simulink model "TEMA"  (R2017a)
settings: Solver=FixedStepAuto  StartTime=0.0  StopTime=10.0  FixedStep=0.01  RelTol=1e-3
libraries: MyEma x1
settings Model: Creator=alexandr.lanin  LastModifiedBy=alexandr.lanin

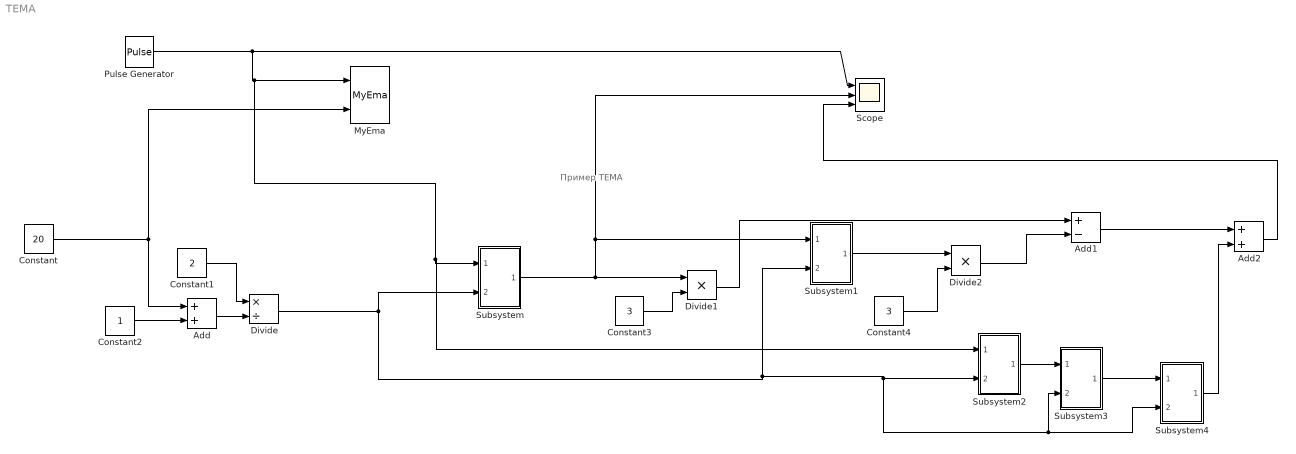
== system TEMA ==
  note: Пример TEMA
  Add : Sum
  Add1 : Sum  Inputs=+-
  Add2 : Sum
  Constant : Constant  Value=20
  Constant1 : Constant  Value=2
  Constant2 : Constant
  Constant3 : Constant  Value=3
  Constant4 : Constant  Value=3
  Divide : Product  Inputs=*/
  Divide1 : Product  Inputs=**
  Divide2 : Product  Inputs=**
  MyEma : MyEma/MyEma
  Pulse Generator : DiscretePulseGenerator  PulseType=Time based  PulseWidth=50
  Scope : Scope  NumInputPorts=3
  Subsystem : Subsystem
  Subsystem1 : Subsystem
  Subsystem2 : Subsystem
  Subsystem3 : Subsystem
  Subsystem4 : Subsystem
  wires:
  Pulse Generator/1 -> Scope/1, Subsystem2/1(In1), Subsystem/1(In1), MyEma/1
  Constant2/1 -> Add/2
  Constant/1 -> MyEma/2, Add/1
  Add/1 -> Divide/2
  Constant1/1 -> Divide/1
  Constant3/1 -> Divide1/2
  Subsystem/1(Out1) -> Divide1/1, Scope/2, Subsystem1/1(In1)
  Subsystem1/1(Out1) -> Divide2/1
  Constant4/1 -> Divide2/2
  Divide2/1 -> Add1/2
  Subsystem3/1(Out1) -> Subsystem4/1(In1)
  Subsystem2/1(Out1) -> Subsystem3/1(In1)
  Divide/1 -> Subsystem/2(In2), Subsystem3/2(In2), Subsystem4/2(In2), Subsystem2/2(In2), Subsystem1/2(In2)
  Add1/1 -> Add2/1
  Subsystem4/1(Out1) -> Add2/2
  Add2/1 -> Scope/3
  Divide1/1 -> Add1/1

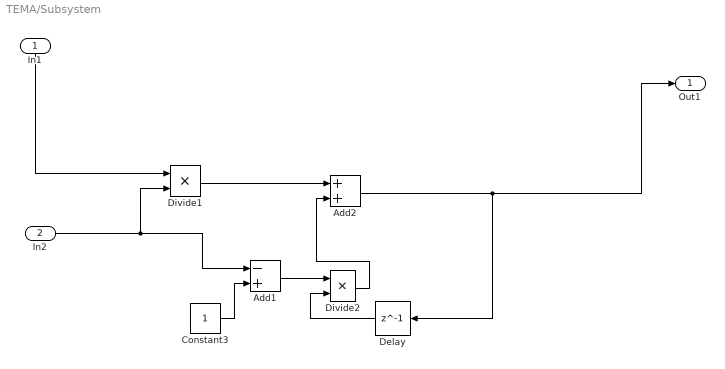
== system TEMA/Subsystem ==
  In1 : Inport
  In2 : Inport  Port=2
  Add1 : Sum  Inputs=-+
  Add2 : Sum
  Constant3 : Constant
  Delay : Delay  DelayLength=1  InitialCondition=0
  Divide1 : Product  Inputs=**
  Divide2 : Product  Inputs=**
  Out1 : Outport
  wires:
  In1/1 -> Divide1/1
  In2/1 -> Add1/1, Divide1/2
  Constant3/1 -> Add1/2
  Divide1/1 -> Add2/1
  Add2/1 -> Out1/1, Delay/1
  Add1/1 -> Divide2/1
  Divide2/1 -> Add2/2
  Delay/1 -> Divide2/2

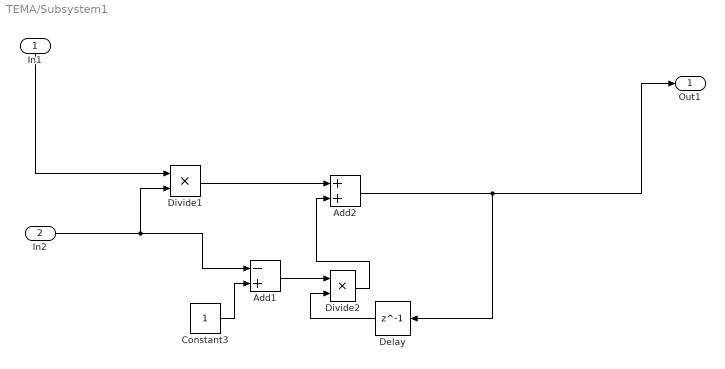
== system TEMA/Subsystem1 ==
  In1 : Inport
  In2 : Inport  Port=2
  Add1 : Sum  Inputs=-+
  Add2 : Sum
  Constant3 : Constant
  Delay : Delay  DelayLength=1  InitialCondition=0
  Divide1 : Product  Inputs=**
  Divide2 : Product  Inputs=**
  Out1 : Outport
  wires:
  In1/1 -> Divide1/1
  In2/1 -> Add1/1, Divide1/2
  Constant3/1 -> Add1/2
  Divide1/1 -> Add2/1
  Add2/1 -> Out1/1, Delay/1
  Add1/1 -> Divide2/1
  Divide2/1 -> Add2/2
  Delay/1 -> Divide2/2

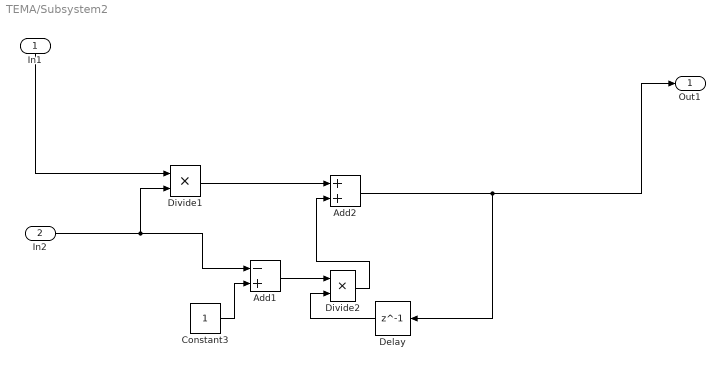
== system TEMA/Subsystem2 ==
  In1 : Inport
  In2 : Inport  Port=2
  Add1 : Sum  Inputs=-+
  Add2 : Sum
  Constant3 : Constant
  Delay : Delay  DelayLength=1  InitialCondition=0
  Divide1 : Product  Inputs=**
  Divide2 : Product  Inputs=**
  Out1 : Outport
  wires:
  In1/1 -> Divide1/1
  In2/1 -> Add1/1, Divide1/2
  Constant3/1 -> Add1/2
  Divide1/1 -> Add2/1
  Add2/1 -> Out1/1, Delay/1
  Add1/1 -> Divide2/1
  Divide2/1 -> Add2/2
  Delay/1 -> Divide2/2

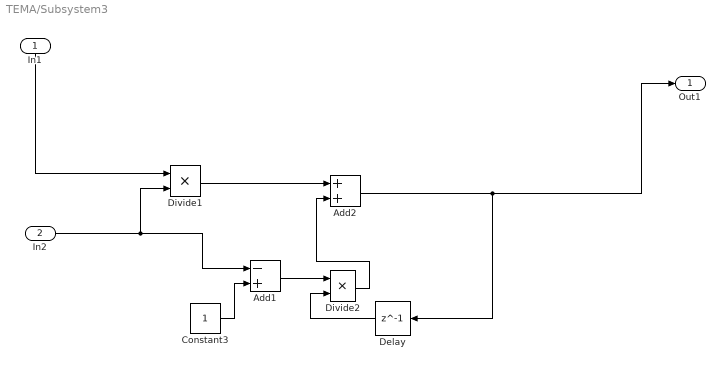
== system TEMA/Subsystem3 ==
  In1 : Inport
  In2 : Inport  Port=2
  Add1 : Sum  Inputs=-+
  Add2 : Sum
  Constant3 : Constant
  Delay : Delay  DelayLength=1  InitialCondition=0
  Divide1 : Product  Inputs=**
  Divide2 : Product  Inputs=**
  Out1 : Outport
  wires:
  In1/1 -> Divide1/1
  In2/1 -> Add1/1, Divide1/2
  Constant3/1 -> Add1/2
  Divide1/1 -> Add2/1
  Add2/1 -> Out1/1, Delay/1
  Add1/1 -> Divide2/1
  Divide2/1 -> Add2/2
  Delay/1 -> Divide2/2

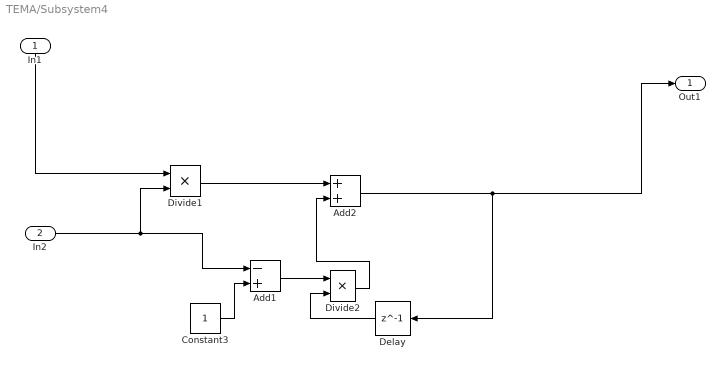
== system TEMA/Subsystem4 ==
  In1 : Inport
  In2 : Inport  Port=2
  Add1 : Sum  Inputs=-+
  Add2 : Sum
  Constant3 : Constant
  Delay : Delay  DelayLength=1  InitialCondition=0
  Divide1 : Product  Inputs=**
  Divide2 : Product  Inputs=**
  Out1 : Outport
  wires:
  In1/1 -> Divide1/1
  In2/1 -> Add1/1, Divide1/2
  Constant3/1 -> Add1/2
  Divide1/1 -> Add2/1
  Add2/1 -> Out1/1, Delay/1
  Add1/1 -> Divide2/1
  Divide2/1 -> Add2/2
  Delay/1 -> Divide2/2
